simulink model "SpringMassPendulumSystem"  (R2024a)
settings: Solver=ode45  StartTime=0.0  StopTime=10.0  RelTol=1e-10
settings Model: Creator=tsarg  LastModifiedBy=tsarg

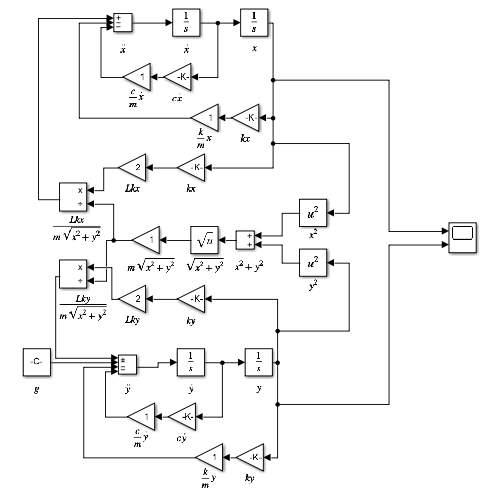
[thumbnail: Simulink's stored preview of the top-level diagram]
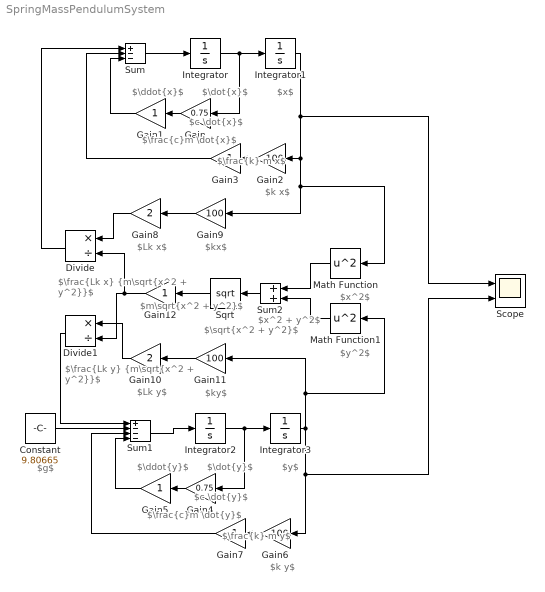
== system SpringMassPendulumSystem ==
  note: $kx$
  note: $x^2 + y^2$
  note: $g$
  note: $\ddot{x}$
  note: $\dot{x}$
  note: $x$
  note: $c \dot{x}$
  note: $\frac{c}m \dot{x}$
  note: $k x$
  note: $\frac{k} m x$
  note: $y$
  note: $\dot{y}$
  note: $c \dot{y}$
  note: $\frac{c}m \dot{y}$
  note: $\ddot{y}$
  note: $k y$
  note: $\frac{k} m y$
  note: $\sqrt{x^2 + y^2}$
  note: $Lk x$
  note: $ky$
  note: $Lk y$
  note: $\frac{Lk x} {m\sqrt{x^2 + y^2}}$
  note: $m\sqrt{x^2 + y^2}$
  note: $\frac{Lk y} {m\sqrt{x^2 + y^2}}$
  note: $x^2$
  note: $y^2$
  Constant : Constant  Value=9.80665
  Divide : Product  Inputs=*/
  Divide1 : Product  Inputs=*/
  Gain : Gain  Gain=0.75
  Gain{1,3,5,7,12} (5 alike) : Gain
  Gain10 : Gain  Gain=2
  Gain{2,6,9,11} (4 alike) : Gain  Gain=100
  Gain4 : Gain  Gain=0.75
  Gain8 : Gain  Gain=2
  Integrator : Integrator  InitialCondition=7
  Integrator1 : Integrator
  Integrator2 : Integrator
  Integrator3 : Integrator  InitialCondition=4
  Math Function : Math  Operator=square
  Math Function1 : Math  Operator=square
  Scope : Scope  NumInputPorts=2
  Sqrt : Sqrt
  Sum : Sum  Inputs=+--
  Sum1 : Sum  Inputs=+---
  Sum2 : Sum
  wires:
  Integrator/1 -> Gain/1, Integrator1/1
  Sum/1 -> Integrator/1
  Gain/1 -> Gain1/1
  Gain2/1 -> Gain3/1
  Gain1/1 -> Sum/3
  Gain3/1 -> Sum/2
  Sum1/1 -> Integrator2/1
  Gain4/1 -> Gain5/1
  Gain7/1 -> Sum1/3
  Integrator2/1 -> Gain4/1, Integrator3/1
  Gain5/1 -> Sum1/4
  Gain6/1 -> Gain7/1
  Constant/1 -> Sum1/2
  Sum2/1 -> Sqrt/1
  Gain10/1 -> Divide1/1
  Gain8/1 -> Divide/1
  Gain9/1 -> Gain8/1
  Gain11/1 -> Gain10/1
  Divide1/1 -> Sum1/1
  Divide/1 -> Sum/1
  Sqrt/1 -> Gain12/1
  Gain12/1 -> Divide1/2, Divide/2
  Integrator1/1 -> Scope/1, Math Function/1, Gain9/1, Gain2/1
  Integrator3/1 -> Scope/2, Gain6/1, Math Function1/1, Gain11/1
  Math Function/1 -> Sum2/1
  Math Function1/1 -> Sum2/2
